simulink model "subcriber"  (R2015a)
settings: Solver=ode3  StartTime=0.0  StopTime=inf  FixedStep=0.01  RelTol=1e-3
model workspace (MAT data in the model file):
  SL_ROS_VariableLengthArrays_MaxSizes.CommonInfo.ArrayTruncateAction = 'EmitWarning'
  SL_ROS_VariableLengthArrays_MaxSizes.MsgTypeMap = containers.Map
  SL_ROS_VariableLengthArrays_MaxSizes.MsgTypeMap.serialization.keys = {'simulator_msgs/Sensor'}
  SL_ROS_VariableLengthArrays_MaxSizes.MsgTypeMap.serialization.values{1}(1).PropertyName = 'Name'
  SL_ROS_VariableLengthArrays_MaxSizes.MsgTypeMap.serialization.values{1}(1).DataType = 'uint8'
  SL_ROS_VariableLengthArrays_MaxSizes.MsgTypeMap.serialization.values{1}(1).MaxLength = 128
  SL_ROS_VariableLengthArrays_MaxSizes.MsgTypeMap.serialization.values{1}(2).PropertyName = 'Values'
  SL_ROS_VariableLengthArrays_MaxSizes.MsgTypeMap.serialization.values{1}(2).DataType = 'double'
  SL_ROS_VariableLengthArrays_MaxSizes.MsgTypeMap.serialization.values{1}(2).MaxLength = 20
  SL_ROS_VariableLengthArrays_MaxSizes.MsgTypeMap.serialization.uniformity = 0
  SL_ROS_VariableLengthArrays_MaxSizes.MsgTypeMap.serialization.keyType = 'char'
  SL_ROS_VariableLengthArrays_MaxSizes.MsgTypeMap.serialization.valueType = 'any'
libraries: realtime_pacer_lib x2, robotlib x1
settings Model: Creator=rblan  LastModifiedBy=rblan

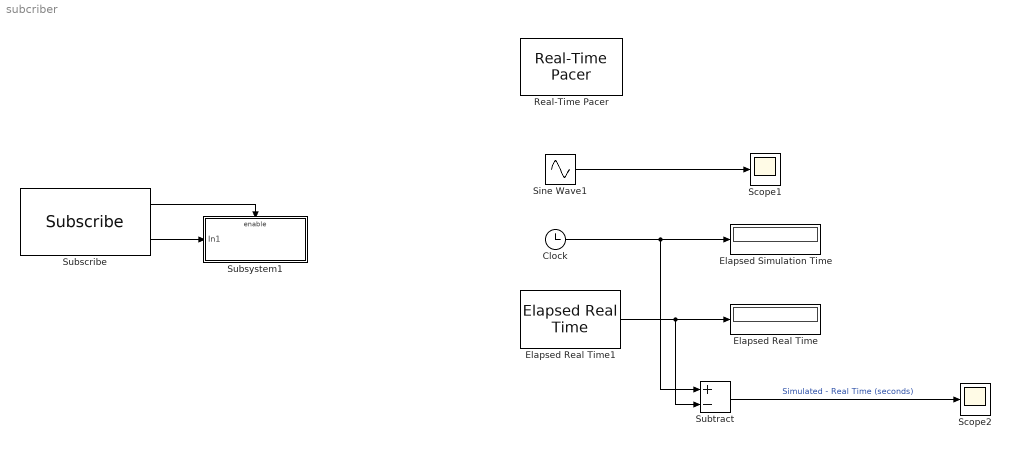
== system subcriber ==
  Clock : Clock
  Elapsed Real Time : Display
      settings: Decimation=2
  Elapsed Real Time1 : realtime_pacer_lib/Elapsed Real Time
  Elapsed Simulation Time : Display
      settings: Decimation=2
  Real-Time Pacer : realtime_pacer_lib/Real-Time Pacer  simTimePerRealTime=inf
  Scope1 : Scope
  Scope2 : Scope
      settings: YMin=-0.08  YMax=-0.01
  Sine Wave1 : Sin  Frequency=2*pi*0.5  SampleTime=0
  Subscribe : robotlib/Subscribe  SourceLibraryInfo=This block requires Robotics System Toolbox  topicSource=Select from ROS network  topic=/Estados  messageType=simulator_msgs/Sensor  sampleTime=-1  messageQueueLength=1
  Subsystem1 : Subsystem
  Subtract : Sum  Inputs=+-
  wires:
  Subscribe/2 -> Subsystem1/1(In1)
  Subscribe/1 -> Subsystem1/Enable
  Clock/1 -> Subtract/1, Elapsed Simulation Time/1
  Sine Wave1/1 -> Scope1/1
  Subtract/1 -> Scope2/1  "Simulated - Real Time (seconds)"
  Elapsed Real Time1/1 -> Subtract/2, Elapsed Real Time/1

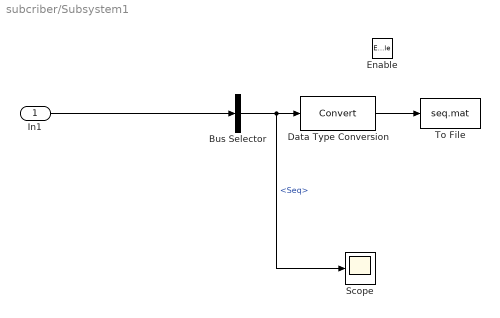
== system subcriber/Subsystem1 ==
  In1 : Inport
  Enable : EnablePort
  Bus Selector : BusSelector  OutputSignals=Header.Seq
  Data Type Conversion : DataTypeConversion
  Scope : Scope
      settings: YMin=800  YMax=1275  SaveName=seqSimulink
  To File : ToFile  Filename=seq.mat  MatrixName=data
  wires:
  Bus Selector/1 -> Scope/1, Data Type Conversion/1  "<Seq>"
  Data Type Conversion/1 -> To File/1
  In1/1 -> Bus Selector/1
